simulink model "System_InvDynamics"  (R2016a)
settings: Solver=VariableStepAuto  StartTime=0.0  StopTime=10  FixedStep=.001  MaxStep=.001  RelTol=1e-6
undefined symbols (not defined in the file or in its folder): Kd, Kp, target
(part 4 of 4)

== matlab function System_InvDynamics/MATLAB Function ==
  data: theta input; theta_ddot input; torque output; theta_dot input
function torque = newton_euler( theta, theta_ddot, theta_dot )
%#codegen
coder.extrinsic('evalin');
coder.extrinsic('newtonEuler');

persistent linkList boundry_conditions;

if isempty(linkList)
    linkList = evalin('base','linkList');
    boundry_conditions.base_angular_velocity = [0;0;0];
    boundry_conditions.base_angular_acceleration = [0;0;0];
    boundry_conditions.base_linear_acceleration = [0;0;9.8];
    boundry_conditions.distal_force = [0;0;0];
    boundry_conditions.distal_torque = [0;0;0];
end

torque = zeros(6,1);
torque = newtonEuler(linkList,theta,theta_dot,theta_ddot,boundry_conditions);


end

== matlab function System_InvDynamics/ABB Arm Dynamics/Laser Tracking ==
  data: theta input; pose output
function pose = laserTracker(theta)
%#codegen
coder.extrinsic('evalin');
persistent Sim_Exact;

if isempty(Sim_Exact)
    Sim_Exact = evalin('base','Sim_Exact');
end


th1 = theta(1);
th2 = theta(2);
th3 = theta(3);
th4 = theta(4);
th5 = theta(5);
th6 = theta(6);


if(Sim_Exact)
    pose = [ sin(th6)*(cos(th4)*sin(th1) + sin(th4)*(cos(th1)*sin(th2)*sin(th3) - cos(th1)*cos(th2)*cos(th3))) + cos(th6)*(cos(th5)*(sin(th1)*sin(th4) - cos(th4)*(cos(th1)*sin(th2)*sin(th3) - cos(th1)*cos(th2)*cos(th3))) - sin(th5)*(cos(th1)*cos(th2)*sin(th3) + cos(th1)*cos(th3)*sin(th2))), cos(th6)*(cos(th4)*sin(th1) + sin(th4)*(cos(th1)*sin(th2)*sin(th3) - cos(th1)*cos(th2)*cos(th3))) - sin(th6)*(cos(th5)*(sin(th1)*sin(th4) - cos(th4)*(cos(th1)*sin(th2)*sin(th3) - cos(th1)*cos(th2)*cos(th3))) - sin(th5)*(cos(th1)*cos(th2)*sin(th3) + cos(th1)*cos(th3)*sin(th2))), - sin(th5)*(sin(th1)*sin(th4) - cos(th4)*(cos(th1)*sin(th2)*sin(th3) - cos(th1)*cos(th2)*cos(th3))) - cos(th5)*(cos(th1)*cos(th2)*sin(th3) + cos(th1)*cos(th3)*sin(th2)), (27*cos(th1)*cos(th2))/100 - (9*sin(th5)*(sin(th1)*sin(th4) - cos(th4)*(cos(th1)*sin(th2)*sin(th3) - cos(th1)*cos(th2)*cos(th3))))/125 - (9*cos(th5)*(cos(th1)*cos(th2)*sin(th3) + cos(th1)*cos(th3)*sin(th2)))/125 - (7*cos(th1)*sin(th2)*sin(th3))/100 + (7*cos(th1)*cos(th2)*cos(th3))/100 - (151*cos(th1)*cos(th2)*sin(th3))/500 - (151*cos(th1)*cos(th3)*sin(th2))/500;
        - sin(th6)*(cos(th1)*cos(th4) - sin(th4)*(sin(th1)*sin(th2)*sin(th3) - cos(th2)*cos(th3)*sin(th1))) - cos(th6)*(cos(th5)*(cos(th1)*sin(th4) + cos(th4)*(sin(th1)*sin(th2)*sin(th3) - cos(th2)*cos(th3)*sin(th1))) + sin(th5)*(cos(th2)*sin(th1)*sin(th3) + cos(th3)*sin(th1)*sin(th2))), sin(th6)*(cos(th5)*(cos(th1)*sin(th4) + cos(th4)*(sin(th1)*sin(th2)*sin(th3) - cos(th2)*cos(th3)*sin(th1))) + sin(th5)*(cos(th2)*sin(th1)*sin(th3) + cos(th3)*sin(th1)*sin(th2))) - cos(th6)*(cos(th1)*cos(th4) - sin(th4)*(sin(th1)*sin(th2)*sin(th3) - cos(th2)*cos(th3)*sin(th1))), sin(th5)*(cos(th1)*sin(th4) + cos(th4)*(sin(th1)*sin(th2)*sin(th3) - cos(th2)*cos(th3)*sin(th1))) - cos(th5)*(cos(th2)*sin(th1)*sin(th3) + cos(th3)*sin(th1)*sin(th2)), (27*cos(th2)*sin(th1))/100 + (9*sin(th5)*(cos(th1)*sin(th4) + cos(th4)*(sin(th1)*sin(th2)*sin(th3) - cos(th2)*cos(th3)*sin(th1))))/125 - (9*cos(th5)*(cos(th2)*sin(th1)*sin(th3) + cos(th3)*sin(th1)*sin(th2)))/125 - (151*cos(th2)*sin(th1)*sin(th3))/500 - (151*cos(th3)*sin(th1)*sin(th2))/500 - (7*sin(th1)*sin(th2)*sin(th3))/100 + (7*cos(th2)*cos(th3)*sin(th1))/100;
        sin(th4)*sin(th6)*(cos(th2)*sin(th3) + cos(th3)*sin(th2)) - cos(th6)*(sin(th5)*(cos(th2)*cos(th3) - sin(th2)*sin(th3)) + cos(th4)*cos(th5)*(cos(th2)*sin(th3) + cos(th3)*sin(th2))), sin(th6)*(sin(th5)*(cos(th2)*cos(th3) - sin(th2)*sin(th3)) + cos(th4)*cos(th5)*(cos(th2)*sin(th3) + cos(th3)*sin(th2))) + cos(th6)*sin(th4)*(cos(th2)*sin(th3) + cos(th3)*sin(th2)), cos(th4)*sin(th5)*(cos(th2)*sin(th3) + cos(th3)*sin(th2)) - cos(th5)*(cos(th2)*cos(th3) - sin(th2)*sin(th3)), (151*sin(th2)*sin(th3))/500 - (151*cos(th2)*cos(th3))/500 - (7*cos(th2)*sin(th3))/100 - (7*cos(th3)*sin(th2))/100 - (27*sin(th2))/100 - (9*cos(th5)*(cos(th2)*cos(th3) - sin(th2)*sin(th3)))/125 + (9*cos(th4)*sin(th5)*(cos(th2)*sin(th3) + cos(th3)*sin(th2)))/125 + 29/100;
        0, 0, 0, 1];
else
    
    pose = [ sin(th6)*(cos(th4)*sin(th1) + sin(th4)*(cos(th1)*sin(th2)*sin(th3) - cos(th1)*cos(th2)*cos(th3))) + cos(th6)*(cos(th5)*(sin(th1)*sin(th4) - cos(th4)*(cos(th1)*sin(th2)*sin(th3) - cos(th1)*cos(th2)*cos(th3))) - sin(th5)*(cos(th1)*cos(th2)*sin(th3) + cos(th1)*cos(th3)*sin(th2))), cos(th6)*(cos(th4)*sin(th1) + sin(th4)*(cos(th1)*sin(th2)*sin(th3) - cos(th1)*cos(th2)*cos(th3))) - sin(th6)*(cos(th5)*(sin(th1)*sin(th4) - cos(th4)*(cos(th1)*sin(th2)*sin(th3) - cos(th1)*cos(th2)*cos(th3))) - sin(th5)*(cos(th1)*cos(th2)*sin(th3) + cos(th1)*cos(th3)*sin(th2))), - sin(th5)*(sin(th1)*sin(th4) - cos(th4)*(cos(th1)*sin(th2)*sin(th3) - cos(th1)*cos(th2)*cos(th3))) - cos(th5)*(cos(th1)*cos(th2)*sin(th3) + cos(th1)*cos(th3)*sin(th2)), (151838081588107*cos(th1)*cos(th2))/562949953421312 - (123928564092639*sin(th1))/72057594037927936 - (7184037743251309*cos(th1))/36893488147419103232 - (7330531551818703*cos(th4)*sin(th1))/36893488147419103232 - (5489399374888815*sin(th1)*sin(th4))/9223372036854775808 + (970893499285375*cos(th5)*(sin(th1)*sin(th4) - cos(th4)*(cos(th1)*sin(th2)*sin(th3) - cos(th1)*cos(th2)*cos(th3))))/9223372036854775808 - (5192391675427195*sin(th5)*(sin(th1)*sin(th4) - cos(th4)*(cos(th1)*sin(th2)*sin(th3) - cos(th1)*cos(th2)*cos(th3))))/72057594037927936 + (1663072680156839*sin(th6)*(cos(th4)*sin(th1) + sin(th4)*(cos(th1)*sin(th2)*sin(th3) - cos(th1)*cos(th2)*cos(th3))))/2305843009213693952 + (1663072680156839*cos(th6)*(cos(th5)*(sin(th1)*sin(th4) - cos(th4)*(cos(th1)*sin(th2)*sin(th3) - cos(th1)*cos(th2)*cos(th3))) - sin(th5)*(cos(th1)*cos(th2)*sin(th3) + cos(th1)*cos(th3)*sin(th2))))/2305843009213693952 + (5489399374888815*cos(th4)*(cos(th1)*sin(th2)*sin(th3) - cos(th1)*cos(th2)*cos(th3)))/9223372036854775808 - (5192391675427195*cos(th5)*(cos(th1)*cos(th2)*sin(th3) + cos(th1)*cos(th3)*sin(th2)))/72057594037927936 - (7330531551818703*sin(th4)*(cos(th1)*sin(th2)*sin(th3) - cos(th1)*cos(th2)*cos(th3)))/36893488147419103232 - (970893499285375*sin(th5)*(cos(th1)*cos(th2)*sin(th3) + cos(th1)*cos(th3)*sin(th2)))/9223372036854775808 - (1259578569946919*cos(th1)*sin(th2)*sin(th3))/18014398509481984 + (1259578569946919*cos(th1)*cos(th2)*cos(th3))/18014398509481984 - (5430591396830085*cos(th1)*cos(th2)*sin(th3))/18014398509481984 - (5430591396830085*cos(th1)*cos(th3)*sin(th2))/18014398509481984;
        - sin(th6)*(cos(th1)*cos(th4) - sin(th4)*(sin(th1)*sin(th2)*sin(th3) - cos(th2)*cos(th3)*sin(th1))) - cos(th6)*(cos(th5)*(cos(th1)*sin(th4) + cos(th4)*(sin(th1)*sin(th2)*sin(th3) - cos(th2)*cos(th3)*sin(th1))) + sin(th5)*(cos(th2)*sin(th1)*sin(th3) + cos(th3)*sin(th1)*sin(th2))), sin(th6)*(cos(th5)*(cos(th1)*sin(th4) + cos(th4)*(sin(th1)*sin(th2)*sin(th3) - cos(th2)*cos(th3)*sin(th1))) + sin(th5)*(cos(th2)*sin(th1)*sin(th3) + cos(th3)*sin(th1)*sin(th2))) - cos(th6)*(cos(th1)*cos(th4) - sin(th4)*(sin(th1)*sin(th2)*sin(th3) - cos(th2)*cos(th3)*sin(th1))), sin(th5)*(cos(th1)*sin(th4) + cos(th4)*(sin(th1)*sin(th2)*sin(th3) - cos(th2)*cos(th3)*sin(th1))) - cos(th5)*(cos(th2)*sin(th1)*sin(th3) + cos(th3)*sin(th1)*sin(th2)), (123928564092639*cos(th1))/72057594037927936 - (7184037743251309*sin(th1))/36893488147419103232 + (7330531551818703*cos(th1)*cos(th4))/36893488147419103232 + (151838081588107*cos(th2)*sin(th1))/562949953421312 + (5489399374888815*cos(th1)*sin(th4))/9223372036854775808 - (970893499285375*cos(th5)*(cos(th1)*sin(th4) + cos(th4)*(sin(th1)*sin(th2)*sin(th3) - cos(th2)*cos(th3)*sin(th1))))/9223372036854775808 + (5192391675427195*sin(th5)*(cos(th1)*sin(th4) + cos(th4)*(sin(th1)*sin(th2)*sin(th3) - cos(th2)*cos(th3)*sin(th1))))/72057594037927936 - (1663072680156839*sin(th6)*(cos(th1)*cos(th4) - sin(th4)*(sin(th1)*sin(th2)*sin(th3) - cos(th2)*cos(th3)*sin(th1))))/2305843009213693952 + (5489399374888815*cos(th4)*(sin(th1)*sin(th2)*sin(th3) - cos(th2)*cos(th3)*sin(th1)))/9223372036854775808 - (5192391675427195*cos(th5)*(cos(th2)*sin(th1)*sin(th3) + cos(th3)*sin(th1)*sin(th2)))/72057594037927936 - (1663072680156839*cos(th6)*(cos(th5)*(cos(th1)*sin(th4) + cos(th4)*(sin(th1)*sin(th2)*sin(th3) - cos(th2)*cos(th3)*sin(th1))) + sin(th5)*(cos(th2)*sin(th1)*sin(th3) + cos(th3)*sin(th1)*sin(th2))))/2305843009213693952 - (7330531551818703*sin(th4)*(sin(th1)*sin(th2)*sin(th3) - cos(th2)*cos(th3)*sin(th1)))/36893488147419103232 - (970893499285375*sin(th5)*(cos(th2)*sin(th1)*sin(th3) + cos(th3)*sin(th1)*sin(th2)))/9223372036854775808 - (5430591396830085*cos(th2)*sin(th1)*sin(th3))/18014398509481984 - (5430591396830085*cos(th3)*sin(th1)*sin(th2))/18014398509481984 - (1259578569946919*sin(th1)*sin(th2)*sin(th3))/18014398509481984 + (1259578569946919*cos(th2)*cos(th3)*sin(th1))/18014398509481984;
        sin(th4)*sin(th6)*(cos(th2)*sin(th3) + cos(th3)*sin(th2)) - cos(th6)*(sin(th5)*(cos(th2)*cos(th3) - sin(th2)*sin(th3)) + cos(th4)*cos(th5)*(cos(th2)*sin(th3) + cos(th3)*sin(th2))), sin(th6)*(sin(th5)*(cos(th2)*cos(th3) - sin(th2)*sin(th3)) + cos(th4)*cos(th5)*(cos(th2)*sin(th3) + cos(th3)*sin(th2))) + cos(th6)*sin(th4)*(cos(th2)*sin(th3) + cos(th3)*sin(th2)), cos(th4)*sin(th5)*(cos(th2)*sin(th3) + cos(th3)*sin(th2)) - cos(th5)*(cos(th2)*cos(th3) - sin(th2)*sin(th3)), (5430591396830085*sin(th2)*sin(th3))/18014398509481984 - (5430591396830085*cos(th2)*cos(th3))/18014398509481984 - (1259578569946919*cos(th2)*sin(th3))/18014398509481984 - (1259578569946919*cos(th3)*sin(th2))/18014398509481984 - (1663072680156839*cos(th6)*(sin(th5)*(cos(th2)*cos(th3) - sin(th2)*sin(th3)) + cos(th4)*cos(th5)*(cos(th2)*sin(th3) + cos(th3)*sin(th2))))/2305843009213693952 - (151838081588107*sin(th2))/562949953421312 + (5489399374888815*cos(th4)*(cos(th2)*sin(th3) + cos(th3)*sin(th2)))/9223372036854775808 - (5192391675427195*cos(th5)*(cos(th2)*cos(th3) - sin(th2)*sin(th3)))/72057594037927936 - (7330531551818703*sin(th4)*(cos(th2)*sin(th3) + cos(th3)*sin(th2)))/36893488147419103232 - (970893499285375*sin(th5)*(cos(th2)*cos(th3) - sin(th2)*sin(th3)))/9223372036854775808 - (970893499285375*cos(th4)*cos(th5)*(cos(th2)*sin(th3) + cos(th3)*sin(th2)))/9223372036854775808 + (5192391675427195*cos(th4)*sin(th5)*(cos(th2)*sin(th3) + cos(th3)*sin(th2)))/72057594037927936 + (1663072680156839*sin(th4)*sin(th6)*(cos(th2)*sin(th3) + cos(th3)*sin(th2)))/2305843009213693952 + 325695105792877/1125899906842624;
        0, 0, 0, 1];
end

== matlab function System_InvDynamics/Trajectory Generator ==
  data: time input; Pos output; Quat output; Vel_des output; Accel_des output
function [Pos, Quat, Vel_des, Accel_des] = trajectory_gen( time )
%#codegen
coder.extrinsic('evalin');
coder.extrinsic('constAccelInterp');
coder.extrinsic('cpMap');

persistent trajectory trans_percent;

if isempty(trajectory) || time == 0
    trajectory = evalin('base','trajectory');
    trans_percent = evalin('base','trans_percent');
end
P = zeros(7,1);
V = zeros(7,1);
A = zeros(7,1);
[P,V,A] = constAccelInterp(time,trajectory, trans_percent);

Pos = P(1:3);
Quat = P(4:7);
Vel = V(1:3);
Qdot = V(4:7);
Accel = A(1:3);
Qddot = A(4:7);

AngVel = zeros(3,1);
Ang_Accel = zeros(3,1);


Quat = Quat/norm(Quat);

cp = zeros(3,3);
cp = cpMap(Quat(2:4));
w_from_Qdot = 2*[-Quat(2:4),Quat(1)*eye(3)+cp];
AngVel = w_from_Qdot* Qdot;
Ang_Accel = w_from_Qdot* Qddot;

Vel_des = zeros(6,1);
Accel_des = zeros(6,1);

Vel_des =  [Vel;AngVel];
Accel_des = [Accel;Ang_Accel];


end

== matlab function System_InvDynamics/Error Calculation ==
  data: time input; Pos_des input; error output; Quat_des input; theta_act input
function error  = error_calc( time, Pos_des, Quat_des, theta_act )
%#codegen
coder.extrinsic('evalin');
coder.extrinsic('dhFwdKine');
coder.extrinsic('transError');
coder.extrinsic('quat2Rot');


persistent linkList;

if isempty(linkList) || time == 0
    linkList = evalin('base','linkList');
end

Td = eye(4,4);
Tc = eye(4,4);
Rd = eye(3,3);

Rd = quat2Rot(Quat_des);
Tc = dhFwdKine(linkList,theta_act);
Td = [Rd Pos_des; 0 0 0 1];

error = zeros(6,1);
error = transError(Td,Tc);


end

== matlab function System_InvDynamics/Velocity Jacobian ==
  data: time input; op_space_vel output; paramList input; paramListDot input; Jv_inv output; Jv_dot output
function [op_space_vel, Jv_inv, Jv_dot]  = vel_jacob_contribution(time, paramList, paramListDot)
%#codegen
coder.extrinsic('evalin');
coder.extrinsic('velocityJacobian');

persistent linkList;

if isempty(linkList) || time == 0
    linkList = evalin('base','linkList');
end
Jv = zeros(6,6);
Jv_dot = zeros(6,6);
[Jv, Jv_dot] = velocityJacobian(linkList, paramList, paramListDot );


op_space_vel = zeros(6,1);
op_space_vel = Jv*paramListDot;

Jv_inv = Jv^-1; %% YOU MAY NEED TO CHANGE THIS IF singularity Presents!
end
